simulink model "mainV03_56"  (R2016b)
settings: Solver=FixedStepAuto  StartTime=0.0  StopTime=inf  FixedStep=Ts  MaxStep=0.2  RelTol=1e-2
undefined symbols (not defined in the file): checks, datetime, decyear, delta_e, deltae_degrees, deltafl_degrees, deltafr_degrees, deltar_degrees, deltat_1, deltat_2, deltat_3, deltat_4, deltat_5, Earth, F, ft, groundReaction, initialValues, juliandate, LD, leapyear, Light, m, MIL, Newton, Raphson, s, sigbuilder_block, Ts, WGS84
libraries: simulink x68, aerolibutil x17, aerolibtransform2 x15, simulink_extras x13, aerolibasang x5, aerolib6dofsys x5, aerolib6dof2 x4, aerolibwind2 x3, aerolibbdyn x3, vrlib x3, aerolibconvert2 x3, aerolibactuator x2
(part 7 of 10)

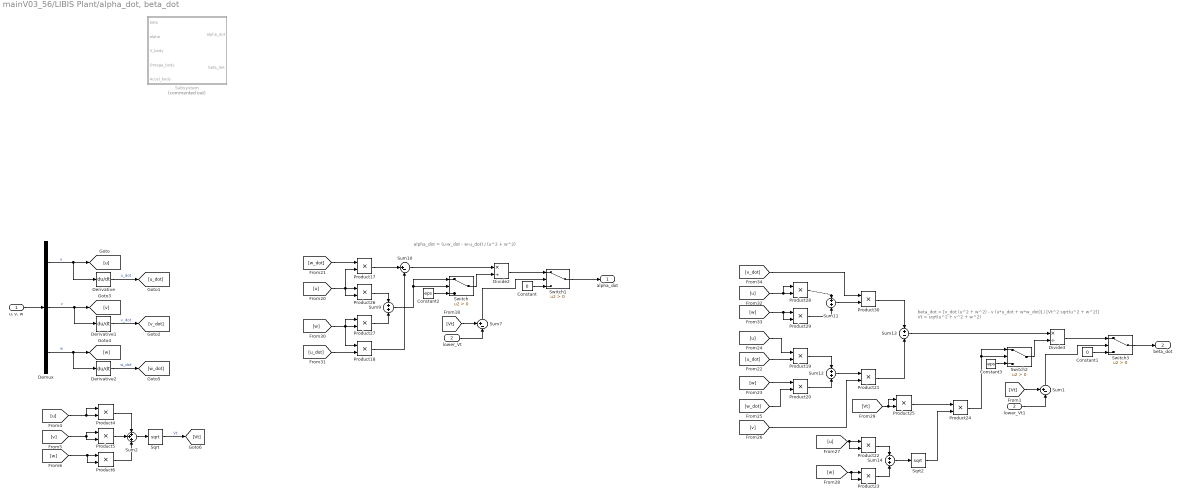
== system mainV03_56/LIBIS Plant/alpha_dot, beta_dot ==
  note: beta_dot = [v_dot (u^2 + w^2) - v (u*u_dot + w*w_dot)] / [Vt^2 sqrt(u^2 + w^2)]
      | Vt = sqrt(u^2 + v^2 + w^2)
  note: alpha_dot = (u·w_dot - w·u_dot) / (u^2 + w^2)
  "u, v, w" : Inport  Unit=meter/s
  lower_Vt : Inport  Port=2
  Constant : Constant  Value=0
  Constant1 : Constant  Value=0
  Constant2 : Constant  Value=eps
  Constant3 : Constant  Value=eps
  Demux : Demux  Outputs=3
  Derivative : Derivative
  Derivative1 : Derivative
  Derivative2 : Derivative
  Divide2 : Product  Inputs=*/
  Divide3 : Product  Inputs=*/
  Product{4..6,17..30} (17 alike) : Product
  Sqrt : Sqrt  SaturateOnIntegerOverflow=on
  Sqrt2 : Sqrt  SaturateOnIntegerOverflow=on
  Subsystem : Subsystem  Commented=on
  Sum1 : Sum  Inputs=+-|
  Sum10 : Sum  Inputs=|+-
  Sum{9,11..12,14} (4 alike) : Sum  Inputs=+|+
  Sum13 : Sum  Inputs=+|-
  Sum2 : Sum  Inputs=+++
  Sum7 : Sum  Inputs=+-|
  Switch{,1..3} (4 alike) : Switch  Criteria=u2 > Threshold
  lower_Vt1 : InportShadow  Port=2
  alpha_dot : Outport  Unit=rad/s
  beta_dot : Outport  Port=2
  wires:
  "u, v, w"/1 -> Demux/1
  Demux/1 -> Derivative/1, [u]  "u"
  Demux/2 -> Derivative1/1, [v]  "v"
  Demux/3 -> Derivative2/1, [w]  "w"
  [u] -> Product4/1, Product4/2
  [w] -> Product6/2, Product6/1
  [v] -> Product5/1, Product5/2
  Product4/1 -> Sum2/1
  Product6/1 -> Sum2/3
  Product5/1 -> Sum2/2
  Sum2/1 -> Sqrt/1
  Sqrt/1 -> [Vt]  "Vt"
  Derivative2/1 -> [w_dot]  "w_dot"
  Derivative/1 -> [u_dot]  "u_dot"
  Derivative1/1 -> [v_dot]  "v_dot"
  Sum7/1 -> Switch1/2
  [Vt] -> Sum7/1
  lower_Vt/1 -> Sum7/2
  [w_dot] -> Product17/1
  [u] -> Product17/2, Product26/2, Product26/1
  [w] -> Product27/1, Product27/2, Product18/1
  [u_dot] -> Product18/2
  Product26/1 -> Sum9/1
  Product27/1 -> Sum9/2
  Product17/1 -> Sum10/1
  Product18/1 -> Sum10/2
  Sum10/1 -> Divide2/1
  [u] -> Product28/1, Product28/2
  [w] -> Product29/2, Product29/1
  Product28/1 -> Sum11/1
  Product29/1 -> Sum11/2
  Sum11/1 -> Product30/2
  [v_dot] -> Product30/1
  [u_dot] -> Product19/2
  [w] -> Product20/1
  Product19/1 -> Sum12/1
  Product20/1 -> Sum12/2
  Sum12/1 -> Product21/1
  [u] -> Product19/1
  [w_dot] -> Product20/2
  [v] -> Product21/2
  Product30/1 -> Sum13/1
  Product21/1 -> Sum13/2
  Sum13/1 -> Divide3/1
  Product22/1 -> Sum14/1
  Product23/1 -> Sum14/2
  [u] -> Product22/2, Product22/1
  [w] -> Product23/2, Product23/1
  [Vt] -> Product25/1, Product25/2
  Product25/1 -> Product24/1
  Sum14/1 -> Sqrt2/1
  Sqrt2/1 -> Product24/2
  Switch/1 -> Divide2/2
  Sum9/1 -> Switch/2, Switch/1
  Constant2/1 -> Switch/3
  Switch2/1 -> Divide3/2
  Product24/1 -> Switch2/2, Switch2/1
  Constant3/1 -> Switch2/3
  Switch3/1 -> beta_dot/1
  Divide2/1 -> Switch1/1
  Switch1/1 -> alpha_dot/1
  Constant/1 -> Switch1/3
  Sum1/1 -> Switch3/2
  Constant1/1 -> Switch3/3
  Divide3/1 -> Switch3/1
  [Vt] -> Sum1/1
  lower_Vt1/1 -> Sum1/2

== system mainV03_56/Pilot Commands/  ==

== system mainV03_56/Pilot Commands/  ==

== system mainV03_56/Pilot Commands/Airspeed Indicator1 ==

== system mainV03_56/Pilot Commands/Altimeter1 ==

== system mainV03_56/Pilot Commands/Artificial Horizon1 ==

== system mainV03_56/Pilot Commands/Buttons to Switches ==
  Buttons : Inport
  Clock : simulink_extras/Flip Flops/Clock  period=2*Ts
  Data Type Conversion : DataTypeConversion  OutDataTypeStr=double
  Data Type Conversion1 : DataTypeConversion  OutDataTypeStr=boolean
  Demux : Demux  Outputs=12
  Hit Crossing : HitCross  HitCrossingOffset=0.5  HitCrossingDirection=rising
  J-K Flip-Flop {1..12} (12 alike) : simulink_extras/Flip Flops/J-K Flip-Flop  initial_condition=0
  Memory : Memory
  Mux : Mux  Inputs=12
  Sum : Sum  Inputs=|++
  Terminator{,1..11} (12 alike) : Terminator
  Switches : Outport
  wires:
  Hit Crossing/1 -> Memory/1, Sum/1
  Buttons/1 -> Data Type Conversion/1
  J-K Flip-Flop 3/2 -> Terminator/1
  Data Type Conversion1/1 -> Demux/1
  Data Type Conversion/1 -> Hit Crossing/1
  Sum/1 -> Data Type Conversion1/1
  Memory/1 -> Sum/2
  J-K Flip-Flop 6/2 -> Terminator1/1
  J-K Flip-Flop 7/2 -> Terminator2/1
  J-K Flip-Flop 10/2 -> Terminator3/1
  J-K Flip-Flop 2/2 -> Terminator4/1
  J-K Flip-Flop 5/2 -> Terminator5/1
  J-K Flip-Flop 8/2 -> Terminator6/1
  J-K Flip-Flop 11/2 -> Terminator7/1
  Clock/1 -> J-K Flip-Flop 9/2, J-K Flip-Flop 12/2, J-K Flip-Flop 4/2, J-K Flip-Flop 1/2, J-K Flip-Flop 2/2, J-K Flip-Flop 5/2, J-K Flip-Flop 11/2, J-K Flip-Flop 8/2, J-K Flip-Flop 3/2, J-K Flip-Flop 10/2, J-K Flip-Flop 7/2, J-K Flip-Flop 6/2
  J-K Flip-Flop 1/2 -> Terminator8/1
  J-K Flip-Flop 4/2 -> Terminator9/1
  J-K Flip-Flop 9/2 -> Terminator10/1
  J-K Flip-Flop 12/2 -> Terminator11/1
  Demux/2 -> J-K Flip-Flop 2/3, J-K Flip-Flop 2/1
  Demux/1 -> J-K Flip-Flop 1/3, J-K Flip-Flop 1/1
  Demux/3 -> J-K Flip-Flop 3/1, J-K Flip-Flop 3/3
  Demux/12 -> J-K Flip-Flop 12/1, J-K Flip-Flop 12/3
  Demux/11 -> J-K Flip-Flop 11/1, J-K Flip-Flop 11/3
  Demux/10 -> J-K Flip-Flop 10/1, J-K Flip-Flop 10/3
  Demux/9 -> J-K Flip-Flop 9/1, J-K Flip-Flop 9/3
  Demux/4 -> J-K Flip-Flop 4/3, J-K Flip-Flop 4/1
  Demux/5 -> J-K Flip-Flop 5/3, J-K Flip-Flop 5/1
  Demux/8 -> J-K Flip-Flop 8/1, J-K Flip-Flop 8/3
  Demux/6 -> J-K Flip-Flop 6/3, J-K Flip-Flop 6/1
  Demux/7 -> J-K Flip-Flop 7/1, J-K Flip-Flop 7/3
  J-K Flip-Flop 1/1 -> Mux/1
  J-K Flip-Flop 12/1 -> Mux/12
  J-K Flip-Flop 11/1 -> Mux/11
  J-K Flip-Flop 10/1 -> Mux/10
  J-K Flip-Flop 9/1 -> Mux/9
  J-K Flip-Flop 8/1 -> Mux/8
  J-K Flip-Flop 7/1 -> Mux/7
  J-K Flip-Flop 4/1 -> Mux/4
  J-K Flip-Flop 5/1 -> Mux/5
  J-K Flip-Flop 6/1 -> Mux/6
  J-K Flip-Flop 2/1 -> Mux/2
  J-K Flip-Flop 3/1 -> Mux/3
  Mux/1 -> Switches/1

== system mainV03_56/Pilot Commands/Climb Rate Indicator1 ==

== system mainV03_56/Pilot Commands/Heading Indicator1 ==

== system mainV03_56/Pilot Commands/If Action Subsystem ==
  Action Port : ActionPort  ActionType=then
  Joystick Input : vrlib/Joystick Input  joyid=1  adjustports=on  forcefeed=off
  Axes : Outport
  Buttons : Outport  Port=2
  wires:
  Joystick Input/1 -> Axes/1
  Joystick Input/2 -> Buttons/1

== system mainV03_56/Pilot Commands/Remaining Capacity Indicator1 ==

== system mainV03_56/Pilot Commands/Signal Builder ==
  Demux : Demux  Tag=STV Demux  Outputs=6
  FromWs : FromWorkspace  Tag=STV FromWs  VariableName=tuvar  SampleTime=0
      SigBuilderData=|
      | common.afterFinalStr = 'Extrapolate'
      | common.sampleTime = 0
      | dataSet.timeRange = [0 500]
      | dataSet.name = 'Group 1'
      | sbobj.Groups.Name = 'Group 1'
      | sbobj.Groups.Signals(1).Name = 'Roll'
      | sbobj.Groups.Signals(1).XData = [0 500]
      | sbobj.Groups.Signals(1).YData = [0 0]
      | sbobj.Groups.Signals(2).Name = 'Pitch'
      | sbobj.Groups.Signals(2).XData = [0 500]
      | sbobj.Groups.Signals(2).YData = [0 0]
      | sbobj.Groups.Signals(3).Name = 'Yaw'
      | sbobj.Groups.Signals(3).XData = [0 500]
      | sbobj.Groups.Signals(3).YData = [0 0]
      | sbobj.Groups.Signals(4).Name = 'Altitude'
      | sbobj.Groups.Signals(4).XData = [0 500]
      | sbobj.Groups.Signals(4).YData = [0 0]
      | sbobj.Groups.Signals(5).Name = 'Throttle1'
      | sbobj.Groups.Signals(5).XData = [0 500]
      | sbobj.Groups.Signals(5).YData = [0 0]
      | sbobj.Groups.Signals(6).Name = 'flightCondition'
      | sbobj.Groups.Signals(6).XData = [0 500]
      | sbobj.Groups.Signals(6).YData = [0 0]
      | sbobj.Groups.TimeRange = [0 500]
  Roll : Outport  Tag=STV Outport
  Pitch : Outport  Tag=STV Outport  Port=2
  Yaw : Outport  Tag=STV Outport  Port=3
  Altitude : Outport  Tag=STV Outport  Port=4
  Throttle1 : Outport  Tag=STV Outport  Port=5
  flightCondition : Outport  Tag=STV Outport  Port=6
  wires:
  FromWs/1 -> Demux/1
  Demux/1 -> Roll/1
  Demux/2 -> Pitch/1
  Demux/3 -> Yaw/1
  Demux/4 -> Altitude/1
  Demux/5 -> Throttle1/1
  Demux/6 -> flightCondition/1

== system mainV03_56/Sensors/Feedthrough Sensors ==
  States : Inport  OutDataTypeStr=Bus: plantDataBus
  Environment : Inport  Port=2  OutDataTypeStr=Bus: envDataBus
  Bus Creator2 : BusCreator  Inputs='LLAMeas','X_nedMeas','VearthMeas','AccelMeas_body','OmegaMeas_body','DCMMeas_body_earth','EulerMeas','VaeroMeas_body','alphaMeas','betaMeas','CGMeas','remainingCapacityMeas'  OutDataTypeStr=Bus: SensorsBus  NonVirtualBus=on
  CPU : Subsystem
  Environment_1 : InportShadow  Port=2  OutDataTypeStr=Bus: envDataBus
  GPS : Subsystem
  IMU : Subsystem
  Pitot : Subsystem
  Veleta : Subsystem
  Sensors : Outport  OutDataTypeStr=Bus: SensorsBus
  wires:
  Environment/1 -> IMU/2(Environment)
  IMU/4(EulerMeas) -> Bus Creator2/7  "EulerMeas"
  Bus Creator2/1 -> Sensors/1  "Sensors"
  CPU/1(CGMeas) -> Bus Creator2/11  "CGMeas"
  GPS/2(X_nedMeas) -> Bus Creator2/2  "X_nedMeas"
  States/1 -> IMU/1(States), GPS/1(States), Pitot/1(States), CPU/1(States), Veleta/1(States)
  IMU/2(OmegaMeas_body) -> Bus Creator2/5  "OmegaMeas_body"
  IMU/1(AccelMeas_body) -> Bus Creator2/4  "AccelMeas_body"
  GPS/1(LLAMeas) -> Bus Creator2/1  "LLAMeas"
  Veleta/1(alphaMeas) -> Bus Creator2/9  "alphaMeas"
  Environment_1/1 -> Pitot/2(Environment)
  Veleta/2(betaMeas) -> Bus Creator2/10  "betaMeas"
  Pitot/1(VaeroMeas_body) -> Bus Creator2/8  "VaeroMeas_body"
  CPU/2(remainingCapacityMeas) -> Bus Creator2/12  "remainingCapacityMeas"
  GPS/3(VearthMeas) -> Bus Creator2/3  "VearthMeas"
  IMU/3(DCMMeas_body_earth) -> Bus Creator2/6  "DCMMeas_body_earth"

== system mainV03_56/Sensors/Noisy Sensors ==
  States : Inport  OutDataTypeStr=Bus: plantDataBus
  Environment : Inport  Port=2  OutDataTypeStr=Bus: envDataBus
  Bus Creator2 : BusCreator  Inputs='LLAMeas','X_nedMeas','VearthMeas','AccelMeas_body','OmegaMeas_body','DCMMeas_body_earth','EulerMeas','VaeroMeas_body','alphaMeas','betaMeas','CGMeas','remainingCapacityMeas'  OutDataTypeStr=Bus: SensorsBus  NonVirtualBus=on
  CPU (Feedthough) : Subsystem
  Environment_1 : InportShadow  Port=2  OutDataTypeStr=Bus: envDataBus
  GPS (Feedthough) : Subsystem
  IMU : Subsystem
  Pitot (Feedthough) : Subsystem
  Veleta (Feedthough) : Subsystem
  Sensors : Outport  OutDataTypeStr=Bus: SensorsBus
  wires:
  Environment/1 -> IMU/2(Environment)
  IMU/4(EulerMeas) -> Bus Creator2/7  "EulerMeas"
  Bus Creator2/1 -> Sensors/1  "Sensors"
  CPU (Feedthough)/1(CGMeas) -> Bus Creator2/11  "CGMeas"
  GPS (Feedthough)/2(X_nedMeas) -> Bus Creator2/2  "X_nedMeas"
  States/1 -> GPS (Feedthough)/1(States), IMU/1(States), Pitot (Feedthough)/1(States), CPU (Feedthough)/1(States), Veleta (Feedthough)/1(States)
  IMU/2(OmegaMeas_body) -> Bus Creator2/5  "OmegaMeas_body"
  IMU/1(AccelMeas_body) -> Bus Creator2/4  "AccelMeas_body"
  GPS (Feedthough)/1(LLAMeas) -> Bus Creator2/1  "LLAMeas"
  Veleta (Feedthough)/1(alphaMeas) -> Bus Creator2/9  "alphaMeas"
  Environment_1/1 -> Pitot (Feedthough)/2(Environment)
  Veleta (Feedthough)/2(betaMeas) -> Bus Creator2/10  "betaMeas"
  Pitot (Feedthough)/1(VaeroMeas_body) -> Bus Creator2/8  "VaeroMeas_body"
  CPU (Feedthough)/2(remainingCapacityMeas) -> Bus Creator2/12  "remainingCapacityMeas"
  GPS (Feedthough)/3(VearthMeas) -> Bus Creator2/3  "VearthMeas"
  IMU/3(DCMMeas_body_earth) -> Bus Creator2/6  "DCMMeas_body_earth"

== system mainV03_56/Visualization/Airspeed Indicator ==

== system mainV03_56/Visualization/Altimeter ==

== system mainV03_56/Visualization/Artificial Horizon ==

== system mainV03_56/Visualization/Axes to VR Axes ==
  Xe : Inport
  Concatenate : Concatenate  NumInputs=3
  Constant : Constant  Value=1.01
  Demux : Demux  Outputs=3
  Sum : Sum  Inputs=|++
  rad-->deg : Gain  Gain=-1  SaturateOnIntegerOverflow=on  OutDataTypeStr=Inherit: Same as input  ParamDataTypeStr=Inherit: Same as input
  rad-->deg1 : Gain  Gain=-1  SaturateOnIntegerOverflow=on  OutDataTypeStr=Inherit: Same as input  ParamDataTypeStr=Inherit: Same as input
  Xe VR : Outport
  wires:
  Xe/1 -> Demux/1
  Concatenate/1 -> Xe VR/1
  rad-->deg1/1 -> Concatenate/2
  rad-->deg/1 -> Concatenate/1
  Demux/1 -> Concatenate/3
  Demux/2 -> rad-->deg/1
  Constant/1 -> Sum/2
  Demux/3 -> Sum/1
  Sum/1 -> rad-->deg1/1

== system mainV03_56/Visualization/Climb Rate Indicator ==

== system mainV03_56/Visualization/Heading Indicator ==

== system mainV03_56/Visualization/Remaining Capacity Indicator ==

== system mainV03_56/Visualization/Subsystem ==
  "X_ned " : Inport
  Euler_angles : Inport  Port=2
  V_body : Inport  Port=3
  V_ned : Inport  Port=4
  Angle Conversion : aerolibconvert2/Angle Conversion  IU=rad  OU=deg
  Angle Conversion1 : aerolibconvert2/Angle Conversion  IU=rad  OU=deg
  Climbrate : Selector  IndexMode=Zero-based  InputPortWidth=3  IndexOptions=Index vector (dialog)  Indices=2  OutputSizes=1
  Concatenate : Concatenate
  Dot Product : DotProduct  SaturateOnIntegerOverflow=on  OutDataTypeStr=Inherit: Inherit via internal rule
  Flightpath Angle : Subsystem
  Heading : Selector  IndexMode=Zero-based  InputPortWidth=3  IndexOptions=Index vector (dialog)  Indices=2  OutputSizes=1
  Height : Selector  IndexMode=Zero-based  InputPortWidth=3  IndexOptions=Index vector (dialog)  Indices=2  OutputSizes=1
  Length Conversion : aerolibconvert2/Length Conversion  IU=m  OU=ft
  Roll Angle : Selector  IndexMode=Zero-based  InputPortWidth=3  IndexOptions=Index vector (dialog)  Indices=0  OutputSizes=1
  Velocity Conversion : aerolibconvert/Velocity Conversion  IU=m/s  OU=kts
  Velocity Conversion1 : aerolibconvert/Velocity Conversion  IU=m/s  OU=ft/s
  rad-->deg1 : Gain  Gain=-1  SaturateOnIntegerOverflow=on  OutDataTypeStr=Inherit: Same as input  ParamDataTypeStr=Inherit: Same as input
  rad-->deg2 : Gain  Gain=-1  SaturateOnIntegerOverflow=on  OutDataTypeStr=Inherit: Same as input  ParamDataTypeStr=Inherit: Same as input
  rad-->deg3 : Gain  Gain=60  SaturateOnIntegerOverflow=on  OutDataTypeStr=Inherit: Same as input  ParamDataTypeStr=Inherit: Same as input
  vt : Sqrt  SaturateOnIntegerOverflow=on
  Airspeed (kts) : Outport
  Height (ft) : Outport  Port=2
  Roll Flightpath (deg) : Outport  Port=3
  Climb Rate (ft/min) : Outport  Port=4
  Heading (deg) : Outport  Port=5
  wires:
  Velocity Conversion1/1 -> rad-->deg3/1
  rad-->deg3/1 -> Climb Rate (ft/min)/1
  V_ned/1 -> Flightpath Angle/1(Ve), Climbrate/1
  Flightpath Angle/1(gamma) -> Concatenate/2
  rad-->deg2/1 -> Velocity Conversion1/1
  Length Conversion/1 -> Height (ft)/1
  Angle Conversion1/1 -> Roll Flightpath (deg)/1
  Height/1 -> rad-->deg1/1
  Angle Conversion/1 -> Heading (deg)/1  "Heading"
  Heading/1 -> Angle Conversion/1
  Velocity Conversion/1 -> Airspeed (kts)/1
  Dot Product/1 -> vt/1
  Roll Angle/1 -> Concatenate/1
  V_body/1 -> Dot Product/2, Dot Product/1
  Concatenate/1 -> Angle Conversion1/1
  vt/1 -> Velocity Conversion/1
  Climbrate/1 -> rad-->deg2/1
  rad-->deg1/1 -> Length Conversion/1
  Euler_angles/1 -> Roll Angle/1, Heading/1
  "X_ned "/1 -> Height/1

== system mainV03_56/Environment/Terrain/Reaction ==
  X : Inport
  V : Inport  Port=2
  -D1 : Gain  Gain=-groundReaction.D
  -K2 : Gain  Gain=-groundReaction.K
  Constant3 : Constant  Value=0
  Constant4 : Constant  Value=0
  Constant5 : Constant  Value=0
  Mux1 : Mux  Inputs=3
  Product1 : Product
  Sel5 : Selector  InputPortWidth=3  IndexOptions=Index vector (dialog)  Indices=3  OutputSizes=1
  Sel6 : Selector  InputPortWidth=3  IndexOptions=Index vector (dialog)  Indices=3  OutputSizes=1
  Sqrt1 : Sqrt  SaturateOnIntegerOverflow=on
  Sum4 : Sum  Inputs=|++
  Sum5 : Sum  Inputs=-+
  Switch3 : Switch  Criteria=u2 > Threshold
  Ze2height1 : UnaryMinus
  Ze_dot2height_dot3 : UnaryMinus
  height2d2 : UnaryMinus
  height2d3 : UnaryMinus
  hground_value1 : Constant  Value=initialValues.href  OutDataTypeStr=double
  hground1 : Outport  Unit=m
  F_earth : Outport  Port=2
  wires:
  Ze2height1/1 -> Sum5/2  "alt"
  X/1 -> Sel6/1
  Sel6/1 -> Ze2height1/1
  Sel5/1 -> Ze_dot2height_dot3/1
  hground_value1/1 -> Sum5/1
  Constant3/1 -> Switch3/1
  Switch3/1 -> height2d2/1
  height2d2/1 -> Sqrt1/1  "d"
  -K2/1 -> Sum4/1
  Product1/1 -> height2d3/1
  height2d3/1 -> Mux1/3
  Sum5/1 -> hground1/1, -K2/1, Switch3/3, Switch3/2  "z"
  Sqrt1/1 -> Product1/1
  Ze_dot2height_dot3/1 -> -D1/1  "z_dot"
  -D1/1 -> Sum4/2
  Sum4/1 -> Product1/2
  V/1 -> Sel5/1
  Mux1/1 -> F_earth/1  "F_earth"
  Constant5/1 -> Mux1/2
  Constant4/1 -> Mux1/1

== system mainV03_56/Environment/Terrain/Reaction1 ==
  X : Inport
  V : Inport  Port=2
  -D1 : Gain  Gain=-groundReaction.D
  -K2 : Gain  Gain=-groundReaction.K
  Constant3 : Constant  Value=0
  Constant4 : Constant  Value=0
  Constant5 : Constant  Value=0
  Mux1 : Mux  Inputs=3
  Product1 : Product
  Sel5 : Selector  InputPortWidth=3  IndexOptions=Index vector (dialog)  Indices=3  OutputSizes=1
  Sel6 : Selector  InputPortWidth=3  IndexOptions=Index vector (dialog)  Indices=3  OutputSizes=1
  Sqrt1 : Sqrt  SaturateOnIntegerOverflow=on
  Sum4 : Sum  Inputs=|++
  Sum5 : Sum  Inputs=-+
  Switch3 : Switch  Criteria=u2 > Threshold
  Ze2height1 : UnaryMinus
  Ze_dot2height_dot3 : UnaryMinus
  height2d2 : UnaryMinus
  height2d3 : UnaryMinus
  hground_value1 : Constant  Value=initialValues.href  OutDataTypeStr=double
  hground1 : Outport  Unit=m
  F_earth : Outport  Port=2
  wires:
  Ze2height1/1 -> Sum5/2  "alt"
  X/1 -> Sel6/1
  Sel6/1 -> Ze2height1/1
  Sel5/1 -> Ze_dot2height_dot3/1
  hground_value1/1 -> Sum5/1
  Constant3/1 -> Switch3/1
  Switch3/1 -> height2d2/1
  height2d2/1 -> Sqrt1/1  "d"
  -K2/1 -> Sum4/1
  Product1/1 -> height2d3/1
  height2d3/1 -> Mux1/3
  Sum5/1 -> hground1/1, -K2/1, Switch3/3, Switch3/2  "z"
  Sqrt1/1 -> Product1/1
  Ze_dot2height_dot3/1 -> -D1/1  "z_dot"
  -D1/1 -> Sum4/2
  Sum4/1 -> Product1/2
  V/1 -> Sel5/1
  Mux1/1 -> F_earth/1  "F_earth"
  Constant5/1 -> Mux1/2
  Constant4/1 -> Mux1/1

== system mainV03_56/Environment/Terrain/Reaction2 ==
  X : Inport
  V : Inport  Port=2
  -D1 : Gain  Gain=-groundReaction.D
  -K2 : Gain  Gain=-groundReaction.K
  Constant3 : Constant  Value=0
  Constant4 : Constant  Value=0
  Constant5 : Constant  Value=0
  Mux1 : Mux  Inputs=3
  Product1 : Product
  Sel5 : Selector  InputPortWidth=3  IndexOptions=Index vector (dialog)  Indices=3  OutputSizes=1
  Sel6 : Selector  InputPortWidth=3  IndexOptions=Index vector (dialog)  Indices=3  OutputSizes=1
  Sqrt1 : Sqrt  SaturateOnIntegerOverflow=on
  Sum4 : Sum  Inputs=|++
  Sum5 : Sum  Inputs=-+
  Switch3 : Switch  Criteria=u2 > Threshold
  Ze2height1 : UnaryMinus
  Ze_dot2height_dot3 : UnaryMinus
  height2d2 : UnaryMinus
  height2d3 : UnaryMinus
  hground_value1 : Constant  Value=initialValues.href  OutDataTypeStr=double
  hground1 : Outport  Unit=m
  F_earth : Outport  Port=2
  wires:
  Ze2height1/1 -> Sum5/2  "alt"
  X/1 -> Sel6/1
  Sel6/1 -> Ze2height1/1
  Sel5/1 -> Ze_dot2height_dot3/1
  hground_value1/1 -> Sum5/1
  Constant3/1 -> Switch3/1
  Switch3/1 -> height2d2/1
  height2d2/1 -> Sqrt1/1  "d"
  -K2/1 -> Sum4/1
  Product1/1 -> height2d3/1
  height2d3/1 -> Mux1/3
  Sum5/1 -> hground1/1, -K2/1, Switch3/3, Switch3/2  "z"
  Sqrt1/1 -> Product1/1
  Ze_dot2height_dot3/1 -> -D1/1  "z_dot"
  -D1/1 -> Sum4/2
  Sum4/1 -> Product1/2
  V/1 -> Sel5/1
  Mux1/1 -> F_earth/1  "F_earth"
  Constant5/1 -> Mux1/2
  Constant4/1 -> Mux1/1

== system mainV03_56/FCS/Fixed-Wing - Cruise/Slider ==

== system mainV03_56/FCS/Fixed-Wing - Cruise/Slider10 ==

== system mainV03_56/FCS/Fixed-Wing - Cruise/Slider11 ==

== system mainV03_56/FCS/Fixed-Wing - Cruise/Slider12 ==

== system mainV03_56/FCS/Fixed-Wing - Cruise/Slider13 ==

== system mainV03_56/FCS/Fixed-Wing - Cruise/Slider6 ==

== system mainV03_56/FCS/Fixed-Wing - Cruise/Slider7 ==

== system mainV03_56/FCS/Fixed-Wing - Cruise/Slider8 ==

== system mainV03_56/FCS/Fixed-Wing - Cruise/Slider9 ==

== system mainV03_56/FCS/Fixed-Wing Climb/Slider ==

== system mainV03_56/FCS/Fixed-Wing Climb/Slider10 ==

== system mainV03_56/FCS/Fixed-Wing Climb/Slider11 ==

== system mainV03_56/FCS/Fixed-Wing Climb/Slider12 ==

== system mainV03_56/FCS/Fixed-Wing Climb/Slider13 ==

== system mainV03_56/FCS/Fixed-Wing Climb/Slider6 ==

== system mainV03_56/FCS/Fixed-Wing Climb/Slider7 ==

== system mainV03_56/FCS/Fixed-Wing Climb/Slider8 ==

== system mainV03_56/FCS/Fixed-Wing Climb/Slider9 ==

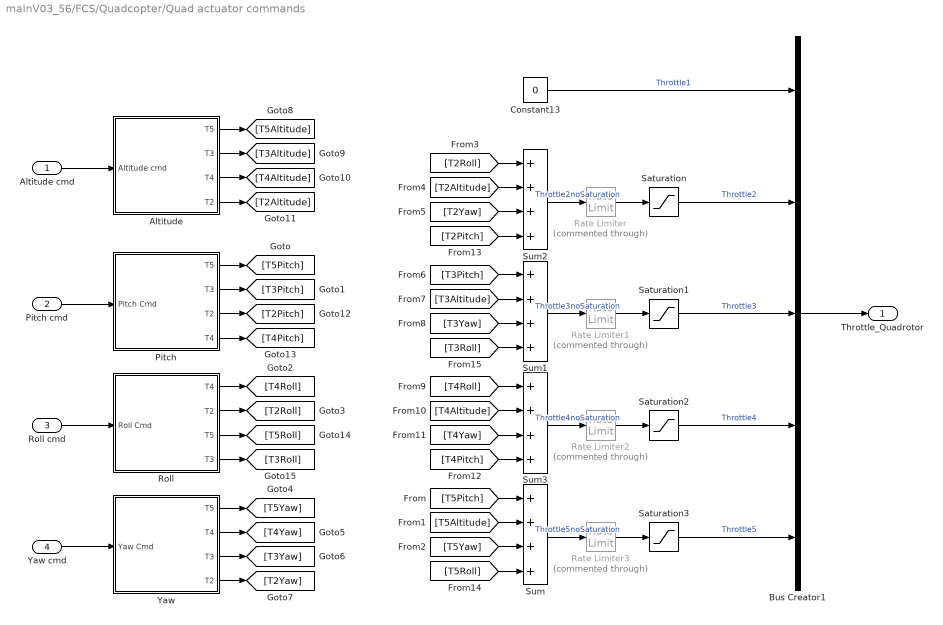
== system mainV03_56/FCS/Quadcopter/Quad actuator commands ==
  Altitude cmd : Inport
  Pitch cmd : Inport  Port=2
  Roll cmd : Inport  Port=3
  Yaw cmd : Inport  Port=4
  Altitude : Subsystem
  Bus Creator1 : BusCreator  Inputs='Throttle1','Throttle2','Throttle3','Throttle4','Throttle5'  OutDataTypeStr=Bus: ThrottleBus  NonVirtualBus=on
  Constant13 : Constant  Value=0
  Pitch : Subsystem
  Rate Limiter{,1..3} (4 alike) : RateLimiter  Commented=through  RisingSlewLimit=0.5  FallingSlewLimit=-0.5  SampleTimeMode=inherited
  Roll : Subsystem
  Saturation{,1..3} (4 alike) : Saturate  UpperLimit=1  LowerLimit=0
  Sum{,1..3} (4 alike) : Sum  Inputs=++++
  Yaw : Subsystem
  Throttle_Quadrotor : Outport  OutDataTypeStr=Bus: ThrottleBus
  wires:
  [T4Yaw] -> Sum3/3
  [T4Altitude] -> Sum3/2
  [T4Roll] -> Sum3/1
  [T3Yaw] -> Sum1/3
  [T3Altitude] -> Sum1/2
  [T3Pitch] -> Sum1/1
  [T2Yaw] -> Sum2/3
  [T2Altitude] -> Sum2/2
  [T2Roll] -> Sum2/1
  [T5Yaw] -> Sum/3
  [T5Altitude] -> Sum/2
  [T5Pitch] -> Sum/1
  Altitude/4(T2) -> [T2Altitude]
  Altitude/3(T4) -> [T4Altitude]
  Altitude/2(T3) -> [T3Altitude]
  Altitude/1(T5) -> [T5Altitude]
  Yaw/4(T2) -> [T2Yaw]
  Yaw/1(T5) -> [T5Yaw]
  Roll/2(T2) -> [T2Roll]
  Roll/1(T4) -> [T4Roll]
  Pitch/2(T3) -> [T3Pitch]
  Pitch/1(T5) -> [T5Pitch]
  Bus Creator1/1 -> Throttle_Quadrotor/1
  Pitch cmd/1 -> Pitch/1(Pitch Cmd)
  Roll cmd/1 -> Roll/1(Roll Cmd)
  Altitude cmd/1 -> Altitude/1(Altitude cmd)
  Yaw/2(T4) -> [T4Yaw]
  Yaw/3(T3) -> [T3Yaw]
  Yaw cmd/1 -> Yaw/1(Yaw Cmd)
  Pitch/3(T2) -> [T2Pitch]
  Pitch/4(T4) -> [T4Pitch]
  [T4Pitch] -> Sum3/4
  [T2Pitch] -> Sum2/4
  Roll/3(T5) -> [T5Roll]
  Roll/4(T3) -> [T3Roll]
  [T5Roll] -> Sum/4
  [T3Roll] -> Sum1/4
  Sum2/1 -> Rate Limiter/1  "Throttle2noSaturation"
  Sum/1 -> Rate Limiter3/1  "Throttle5noSaturation"
  Sum3/1 -> Rate Limiter2/1  "Throttle4noSaturation"
  Sum1/1 -> Rate Limiter1/1  "Throttle3noSaturation"
  Constant13/1 -> Bus Creator1/1  "Throttle1"
  Saturation/1 -> Bus Creator1/2  "Throttle2"
  Saturation1/1 -> Bus Creator1/3  "Throttle3"
  Saturation2/1 -> Bus Creator1/4  "Throttle4"
  Saturation3/1 -> Bus Creator1/5  "Throttle5"
  Rate Limiter/1 -> Saturation/1
  Rate Limiter1/1 -> Saturation1/1
  Rate Limiter2/1 -> Saturation2/1
  Rate Limiter3/1 -> Saturation3/1

== system mainV03_56/FCS/Quadcopter/Slider ==

== system mainV03_56/FCS/Quadcopter/Slider10 ==

== system mainV03_56/FCS/Quadcopter/Slider11 ==

== system mainV03_56/FCS/Quadcopter/Slider12 ==

== system mainV03_56/FCS/Quadcopter/Slider13 ==

== system mainV03_56/FCS/Quadcopter/Slider6 ==

== system mainV03_56/FCS/Quadcopter/Slider7 ==

== system mainV03_56/FCS/Quadcopter/Slider8 ==

== system mainV03_56/FCS/Quadcopter/Slider9 ==

== system mainV03_56/FCS/Quadcopter --> Fixed-Wing/Quad actuator commands ==
  Altitude cmd : Inport
  Pitch cmd : Inport  Port=2
  Roll cmd : Inport  Port=3
  Yaw cmd : Inport  Port=4
  Throttle1 : Inport  Port=5
  Altitude : Subsystem
  Bus Creator1 : BusCreator  Inputs='Throttle1','Throttle2','Throttle3','Throttle4','Throttle5'  OutDataTypeStr=Bus: ThrottleBus  NonVirtualBus=on
  Pitch : Subsystem
  Rate Limiter{,1..3} (4 alike) : RateLimiter  Commented=through  RisingSlewLimit=0.5  FallingSlewLimit=-0.5  SampleTimeMode=inherited
  Roll : Subsystem
  Saturation{,1..3} (4 alike) : Saturate  UpperLimit=1  LowerLimit=0
  Sum{,1..3} (4 alike) : Sum  Inputs=++++
  Yaw : Subsystem
  Throttle_Quadrotor : Outport  OutDataTypeStr=Bus: ThrottleBus
  wires:
  [T4Yaw] -> Sum3/3
  [T4Altitude] -> Sum3/2
  [T4Roll] -> Sum3/1
  [T3Yaw] -> Sum1/3
  [T3Altitude] -> Sum1/2
  [T3Pitch] -> Sum1/1
  [T2Yaw] -> Sum2/3
  [T2Altitude] -> Sum2/2
  [T2Roll] -> Sum2/1
  [T5Yaw] -> Sum/3
  [T5Altitude] -> Sum/2
  [T5Pitch] -> Sum/1
  Altitude/4(T2) -> [T2Altitude]
  Altitude/3(T4) -> [T4Altitude]
  Altitude/2(T3) -> [T3Altitude]
  Altitude/1(T5) -> [T5Altitude]
  Yaw/4(T2) -> [T2Yaw]
  Yaw/1(T5) -> [T5Yaw]
  Roll/2(T2) -> [T2Roll]
  Roll/1(T4) -> [T4Roll]
  Pitch/2(T3) -> [T3Pitch]
  Pitch/1(T5) -> [T5Pitch]
  Bus Creator1/1 -> Throttle_Quadrotor/1
  Pitch cmd/1 -> Pitch/1(Pitch Cmd)
  Roll cmd/1 -> Roll/1(Roll Cmd)
  Altitude cmd/1 -> Altitude/1(Altitude cmd)
  Yaw/2(T4) -> [T4Yaw]
  Yaw/3(T3) -> [T3Yaw]
  Yaw cmd/1 -> Yaw/1(Yaw Cmd)
  Pitch/3(T2) -> [T2Pitch]
  Pitch/4(T4) -> [T4Pitch]
  [T4Pitch] -> Sum3/4
  [T2Pitch] -> Sum2/4
  Roll/3(T5) -> [T5Roll]
  Roll/4(T3) -> [T3Roll]
  [T5Roll] -> Sum/4
  [T3Roll] -> Sum1/4
  Sum2/1 -> Rate Limiter/1  "Throttle2noSaturation"
  Sum/1 -> Rate Limiter3/1  "Throttle5noSaturation"
  Sum3/1 -> Rate Limiter2/1  "Throttle4noSaturation"
  Sum1/1 -> Rate Limiter1/1  "Throttle3noSaturation"
  Throttle1/1 -> Bus Creator1/1  "Throttle1"
  Saturation/1 -> Bus Creator1/2  "Throttle2"
  Saturation1/1 -> Bus Creator1/3  "Throttle3"
  Saturation2/1 -> Bus Creator1/4  "Throttle4"
  Saturation3/1 -> Bus Creator1/5  "Throttle5"
  Rate Limiter/1 -> Saturation/1
  Rate Limiter1/1 -> Saturation1/1
  Rate Limiter2/1 -> Saturation2/1
  Rate Limiter3/1 -> Saturation3/1

== system mainV03_56/FCS/Quadcopter --> Fixed-Wing/Slider10 ==

== system mainV03_56/FCS/Quadcopter --> Fixed-Wing/Slider11 ==

== system mainV03_56/FCS/Quadcopter --> Fixed-Wing/Slider12 ==

== system mainV03_56/FCS/Quadcopter --> Fixed-Wing/Slider13 ==

== system mainV03_56/FCS/Quadcopter --> Fixed-Wing/Slider9 ==

== system mainV03_56/FCS/TakeOff/Slider ==

== system mainV03_56/FCS/TakeOff/Slider10 ==

== system mainV03_56/FCS/TakeOff/Slider11 ==

== system mainV03_56/FCS/TakeOff/Slider12 ==

== system mainV03_56/FCS/TakeOff/Slider13 ==

== system mainV03_56/FCS/TakeOff/Slider6 ==

== system mainV03_56/FCS/TakeOff/Slider7 ==

== system mainV03_56/FCS/TakeOff/Slider8 ==

== system mainV03_56/FCS/TakeOff/Slider9 ==

== system mainV03_56/LIBIS Plant/Aerodynamics/CD ==
  prelook-ups : Inport
  plantData : Inport  Port=2
  actuators : Inport  Port=3
  Add : Sum  Inputs=+++++++
  Bus Selector : BusSelector  OutputSignals=alpha,alpha_dot,Omega_body.q
  Bus Selector1 : BusSelector  OutputSignals=alpha,beta,alt,xcg,deltae,deltar,deltafr,deltafl
  Bus Selector2 : BusSelector  OutputSignals=deltae,deltafr,deltafl
  CD0 : Interpolation_n-D  NumberOfTableDimensions=8  Table=LD.Stability.CD0  ExtrapMethod=Clip  DiagnosticForOutOfRangeInput=Warning  RequireIndexFractionAsBus=on  ValidIndexMayReachLast=on  InternalRulePriority=Speed
      settings: InputPortMap=u0,u1,u2,u3,u4,u5,u6,u7
  CDalpha : Interpolation_n-D  NumberOfTableDimensions=8  Table=LD.Stability.CDalpha  ExtrapMethod=Clip  DiagnosticForOutOfRangeInput=Warning  RequireIndexFractionAsBus=on  ValidIndexMayReachLast=on  InternalRulePriority=Speed
      settings: InputPortMap=u0,u1,u2,u3,u4,u5,u6,u7
  CDalpha_dot : Interpolation_n-D  NumberOfTableDimensions=8  Table=LD.Stability.CDalpha_dot  ExtrapMethod=Clip  RequireIndexFractionAsBus=on  ValidIndexMayReachLast=on  InternalRulePriority=Speed
      settings: InputPortMap=u0,u1,u2,u3,u4,u5,u6,u7
  CDdeltae : Interpolation_n-D  NumberOfTableDimensions=8  Table=LD.Stability.CDdeltae  ExtrapMethod=Clip  RequireIndexFractionAsBus=on  ValidIndexMayReachLast=on  InternalRulePriority=Speed
      settings: InputPortMap=u0,u1,u2,u3,u4,u5,u6,u7
  CDdeltafr : Interpolation_n-D  NumberOfTableDimensions=8  Table=LD.Stability.CDdeltafr  ExtrapMethod=Clip  RequireIndexFractionAsBus=on  ValidIndexMayReachLast=on  InternalRulePriority=Speed
      settings: InputPortMap=u0,u1,u2,u3,u4,u5,u6,u7
  CDdeltafrl : Interpolation_n-D  NumberOfTableDimensions=8  Table=LD.Stability.CDdeltafl  ExtrapMethod=Clip  RequireIndexFractionAsBus=on  ValidIndexMayReachLast=on  InternalRulePriority=Speed
      settings: InputPortMap=u0,u1,u2,u3,u4,u5,u6,u7
  CDq : Interpolation_n-D  NumberOfTableDimensions=8  Table=LD.Stability.CDq  ExtrapMethod=Clip  RequireIndexFractionAsBus=on  ValidIndexMayReachLast=on  InternalRulePriority=Speed
      settings: InputPortMap=u0,u1,u2,u3,u4,u5,u6,u7
  Product{,1..5} (6 alike) : Product
  CD : Outport
  wires:
  prelook-ups/1 -> Bus Selector1/1
  CD0/1 -> Add/1
  Add/1 -> CD/1
  plantData/1 -> Bus Selector/1
  actuators/1 -> Bus Selector2/1
  Product/1 -> Add/2
  Bus Selector/1 -> Product/2  "<alpha>"
  Bus Selector2/1 -> Product3/2  "<deltae>"
  CDdeltae/1 -> Product3/1
  Product3/1 -> Add/5
  Product2/1 -> Add/4
  Product1/1 -> Add/3
  CDalpha_dot/1 -> Product1/1
  CDq/1 -> Product2/1
  Bus Selector/3 -> Product2/2  "<q>"
  Bus Selector/2 -> Product1/2  "<alpha_dot>"
  Bus Selector1/8 -> CD0/8, CDalpha/8, CDq/8, CDdeltafrl/8, CDdeltafr/8, CDdeltae/8, CDalpha_dot/8  "<deltafl>"
  Bus Selector1/7 -> CD0/7, CDalpha/7, CDq/7, CDdeltafrl/7, CDdeltafr/7, CDdeltae/7, CDalpha_dot/7  "<deltafr>"
  Bus Selector1/6 -> CD0/6, CDalpha/6, CDq/6, CDdeltafrl/6, CDdeltafr/6, CDdeltae/6, CDalpha_dot/6  "<deltar>"
  Bus Selector1/5 -> CD0/5, CDalpha/5, CDq/5, CDdeltafrl/5, CDdeltafr/5, CDdeltae/5, CDalpha_dot/5  "<deltae>"
  Bus Selector1/3 -> CD0/3, CDalpha/3, CDq/3, CDdeltafrl/3, CDdeltafr/3, CDdeltae/3, CDalpha_dot/3  "<alt>"
  Bus Selector1/4 -> CD0/4, CDalpha/4, CDq/4, CDdeltafrl/4, CDdeltafr/4, CDdeltae/4, CDalpha_dot/4  "<xcg>"
  Bus Selector1/1 -> CD0/1, CDalpha/1, CDdeltafrl/1, CDdeltafr/1, CDdeltae/1, CDq/1, CDalpha_dot/1  "<alpha>"
  Bus Selector2/3 -> Product5/2  "<deltafl>"
  CDdeltafrl/1 -> Product5/1
  Product5/1 -> Add/7
  Product4/1 -> Add/6
  CDdeltafr/1 -> Product4/1
  Bus Selector2/2 -> Product4/2  "<deltafr>"
  Bus Selector1/2 -> CD0/2, CDdeltafrl/2, CDdeltafr/2, CDdeltae/2, CDq/2, CDalpha_dot/2, CDalpha/2  "<beta>"
  CDalpha/1 -> Product/1

== system mainV03_56/LIBIS Plant/Aerodynamics/CL ==
  prelook-ups : Inport
  plantData : Inport  Port=2
  actuators : Inport  Port=3
  Add1 : Sum  Inputs=+++++++
  Bus Selector2 : BusSelector  OutputSignals=alpha,alpha_dot,Omega_body.q
  Bus Selector4 : BusSelector  OutputSignals=alpha,beta,alt,xcg,deltae,deltar,deltafr,deltafl
  Bus Selector5 : BusSelector  OutputSignals=deltae,deltafr,deltafl
  CL0 : Interpolation_n-D  NumberOfTableDimensions=8  Table=LD.Stability.CL0  RequireIndexFractionAsBus=on  InternalRulePriority=Speed
      settings: InputPortMap=u0,u1,u2,u3,u4,u5,u6,u7
  CLalpha : Interpolation_n-D  NumberOfTableDimensions=8  Table=LD.Stability.CLalpha  ExtrapMethod=Clip  DiagnosticForOutOfRangeInput=Warning  RequireIndexFractionAsBus=on  ValidIndexMayReachLast=on  InternalRulePriority=Speed
      settings: InputPortMap=u0,u1,u2,u3,u4,u5,u6,u7
  CLalpha_dot : Interpolation_n-D  NumberOfTableDimensions=8  Table=LD.Stability.CLalpha_dot  ExtrapMethod=Clip  RequireIndexFractionAsBus=on  ValidIndexMayReachLast=on  InternalRulePriority=Speed
      settings: InputPortMap=u0,u1,u2,u3,u4,u5,u6,u7
  CLdeltae : Interpolation_n-D  NumberOfTableDimensions=8  Table=LD.Stability.CLdeltae  ExtrapMethod=Clip  RequireIndexFractionAsBus=on  ValidIndexMayReachLast=on  InternalRulePriority=Speed
      settings: InputPortMap=u0,u1,u2,u3,u4,u5,u6,u7
  CLdeltafr : Interpolation_n-D  NumberOfTableDimensions=8  Table=LD.Stability.CLdeltafr  ExtrapMethod=Clip  RequireIndexFractionAsBus=on  ValidIndexMayReachLast=on  InternalRulePriority=Speed
      settings: InputPortMap=u0,u1,u2,u3,u4,u5,u6,u7
  CLdeltafrl : Interpolation_n-D  NumberOfTableDimensions=8  Table=LD.Stability.CLdeltafl  ExtrapMethod=Clip  RequireIndexFractionAsBus=on  ValidIndexMayReachLast=on  InternalRulePriority=Speed
      settings: InputPortMap=u0,u1,u2,u3,u4,u5,u6,u7
  CLq : Interpolation_n-D  NumberOfTableDimensions=8  Table=LD.Stability.CLq  ExtrapMethod=Clip  RequireIndexFractionAsBus=on  ValidIndexMayReachLast=on  InternalRulePriority=Speed
      settings: InputPortMap=u0,u1,u2,u3,u4,u5,u6,u7
  Product{6..11} (6 alike) : Product
  CL : Outport
  wires:
  prelook-ups/1 -> Bus Selector4/1
  CL0/1 -> Add1/1
  Add1/1 -> CL/1
  plantData/1 -> Bus Selector2/1
  actuators/1 -> Bus Selector5/1
  Product6/1 -> Add1/2
  Bus Selector2/1 -> Product6/2  "<alpha>"
  Bus Selector5/1 -> Product9/2  "<deltae>"
  CLdeltae/1 -> Product9/1
  Product9/1 -> Add1/5
  Product8/1 -> Add1/4
  Product7/1 -> Add1/3
  CLalpha_dot/1 -> Product7/1
  CLq/1 -> Product8/1
  Bus Selector2/3 -> Product8/2  "<q>"
  Bus Selector2/2 -> Product7/2  "<alpha_dot>"
  Bus Selector4/8 -> CL0/8, CLalpha/8, CLq/8, CLdeltafrl/8, CLdeltafr/8, CLdeltae/8, CLalpha_dot/8  "<deltafl>"
  Bus Selector4/7 -> CL0/7, CLalpha/7, CLq/7, CLdeltafrl/7, CLdeltafr/7, CLdeltae/7, CLalpha_dot/7  "<deltafr>"
  Bus Selector4/6 -> CL0/6, CLalpha/6, CLq/6, CLdeltafrl/6, CLdeltafr/6, CLdeltae/6, CLalpha_dot/6  "<deltar>"
  Bus Selector4/5 -> CL0/5, CLalpha/5, CLq/5, CLdeltafrl/5, CLdeltafr/5, CLdeltae/5, CLalpha_dot/5  "<deltae>"
  Bus Selector4/3 -> CL0/3, CLalpha/3, CLq/3, CLdeltafrl/3, CLdeltafr/3, CLdeltae/3, CLalpha_dot/3  "<alt>"
  Bus Selector4/4 -> CL0/4, CLalpha/4, CLq/4, CLdeltafrl/4, CLdeltafr/4, CLdeltae/4, CLalpha_dot/4  "<xcg>"
  Bus Selector4/1 -> CL0/1, CLalpha/1, CLdeltafrl/1, CLdeltafr/1, CLdeltae/1, CLq/1, CLalpha_dot/1  "<alpha>"
  Bus Selector5/3 -> Product11/2  "<deltafl>"
  CLdeltafrl/1 -> Product11/1
  Product11/1 -> Add1/7
  Product10/1 -> Add1/6
  CLdeltafr/1 -> Product10/1
  Bus Selector5/2 -> Product10/2  "<deltafr>"
  Bus Selector4/2 -> CL0/2, CLdeltafrl/2, CLdeltafr/2, CLdeltae/2, CLq/2, CLalpha_dot/2, CLalpha/2  "<beta>"
  CLalpha/1 -> Product6/1

== system mainV03_56/LIBIS Plant/Aerodynamics/CY ==
  prelook-ups : Inport
  plantData : Inport  Port=2
  actuators : Inport  Port=3
  Add : Sum  Inputs=++++++
  Bus Selector : BusSelector  OutputSignals=beta,Omega_body.p,Omega_body.r
  Bus Selector1 : BusSelector  OutputSignals=alpha,beta,alt,xcg,deltae,deltar,deltafr,deltafl
  Bus Selector2 : BusSelector  OutputSignals=deltar,deltafr,deltafl
  CYbeta : Interpolation_n-D  NumberOfTableDimensions=8  Table=LD.Stability.CYbeta  ExtrapMethod=Clip  RequireIndexFractionAsBus=on  ValidIndexMayReachLast=on  InternalRulePriority=Speed
      settings: InputPortMap=u0,u1,u2,u3,u4,u5,u6,u7
  CYdeltafl : Interpolation_n-D  NumberOfTableDimensions=8  Table=LD.Stability.CYdeltafl  ExtrapMethod=Clip  RequireIndexFractionAsBus=on  ValidIndexMayReachLast=on  InternalRulePriority=Speed
      settings: InputPortMap=u0,u1,u2,u3,u4,u5,u6,u7
  CYdeltafr : Interpolation_n-D  NumberOfTableDimensions=8  Table=LD.Stability.CYdeltafr  ExtrapMethod=Clip  RequireIndexFractionAsBus=on  ValidIndexMayReachLast=on  InternalRulePriority=Speed
      settings: InputPortMap=u0,u1,u2,u3,u4,u5,u6,u7
  "CYdeltar " : Interpolation_n-D  NumberOfTableDimensions=8  Table=LD.Stability.CYdeltar  ExtrapMethod=Clip  RequireIndexFractionAsBus=on  ValidIndexMayReachLast=on  InternalRulePriority=Speed
      settings: InputPortMap=u0,u1,u2,u3,u4,u5,u6,u7
  CYp : Interpolation_n-D  NumberOfTableDimensions=8  Table=LD.Stability.CYp  ExtrapMethod=Clip  RequireIndexFractionAsBus=on  ValidIndexMayReachLast=on  InternalRulePriority=Speed
      settings: InputPortMap=u0,u1,u2,u3,u4,u5,u6,u7
  CYr : Interpolation_n-D  NumberOfTableDimensions=8  Table=LD.Stability.CYr  ExtrapMethod=Clip  RequireIndexFractionAsBus=on  ValidIndexMayReachLast=on  InternalRulePriority=Speed
      settings: InputPortMap=u0,u1,u2,u3,u4,u5,u6,u7
  Product{,1..5} (6 alike) : Product
  CY : Outport
  wires:
  Bus Selector1/8 -> CYbeta/8, CYr/8, "CYdeltar "/8, CYdeltafl/8, CYdeltafr/8, CYp/8  "<deltafl>"
  Bus Selector1/7 -> CYbeta/7, CYr/7, "CYdeltar "/7, CYdeltafl/7, CYdeltafr/7, CYp/7  "<deltafr>"
  Bus Selector1/6 -> CYbeta/6, CYr/6, "CYdeltar "/6, CYdeltafl/6, CYdeltafr/6, CYp/6  "<deltar>"
  prelook-ups/1 -> Bus Selector1/1
  Bus Selector1/5 -> CYbeta/5, CYr/5, "CYdeltar "/5, CYdeltafl/5, CYdeltafr/5, CYp/5  "<deltae>"
  Bus Selector1/3 -> CYbeta/3, CYr/3, "CYdeltar "/3, CYdeltafl/3, CYdeltafr/3, CYp/3  "<alt>"
  Bus Selector1/4 -> CYbeta/4, CYr/4, "CYdeltar "/4, CYdeltafl/4, CYdeltafr/4, CYp/4  "<xcg>"
  Bus Selector1/1 -> CYbeta/1, CYdeltafl/1, CYdeltafr/1, "CYdeltar "/1, CYr/1, CYp/1  "<alpha>"
  Add/1 -> CY/1
  plantData/1 -> Bus Selector/1
  actuators/1 -> Bus Selector2/1
  CYbeta/1 -> Product/1
  Product/1 -> Add/1
  Bus Selector/1 -> Product/2  "<beta>"
  Bus Selector2/1 -> Product3/2  "<deltar>"
  "CYdeltar "/1 -> Product3/1
  Product3/1 -> Add/4
  Product2/1 -> Add/3
  Product1/1 -> Add/2
  CYp/1 -> Product1/1
  CYr/1 -> Product2/1
  Bus Selector/3 -> Product2/2  "<r>"
  Bus Selector/2 -> Product1/2  "<p>"
  CYdeltafl/1 -> Product5/1
  Product5/1 -> Add/6
  Product4/1 -> Add/5
  CYdeltafr/1 -> Product4/1
  Bus Selector2/2 -> Product4/2  "<deltafr>"
  Bus Selector2/3 -> Product5/2  "<deltafl>"
  Bus Selector1/2 -> CYdeltafl/2, CYdeltafr/2, "CYdeltar "/2, CYr/2, CYp/2, CYbeta/2  "<beta>"

== system mainV03_56/LIBIS Plant/Aerodynamics/Cl ==
  prelook-ups1 : Inport
  plantData : Inport  Port=2
  actuators : Inport  Port=3
  Add1 : Sum  Inputs=++++++
  Bus Selector3 : BusSelector  OutputSignals=beta,Omega_body.p,Omega_body.r
  Bus Selector4 : BusSelector  OutputSignals=alpha,beta,alt,xcg,deltae,deltar,deltafr,deltafl
  Bus Selector5 : BusSelector  OutputSignals=deltar,deltafr,deltafl
  Clbeta : Interpolation_n-D  NumberOfTableDimensions=8  Table=LD.Stability.Clbeta  ExtrapMethod=Clip  RequireIndexFractionAsBus=on  ValidIndexMayReachLast=on  InternalRulePriority=Speed
      settings: InputPortMap=u0,u1,u2,u3,u4,u5,u6,u7
  Cldeltafl : Interpolation_n-D  NumberOfTableDimensions=8  Table=LD.Stability.Cldeltafl  ExtrapMethod=Clip  RequireIndexFractionAsBus=on  ValidIndexMayReachLast=on  InternalRulePriority=Speed
      settings: InputPortMap=u0,u1,u2,u3,u4,u5,u6,u7
  Cldeltafr : Interpolation_n-D  NumberOfTableDimensions=8  Table=LD.Stability.Cldeltafr  ExtrapMethod=Clip  RequireIndexFractionAsBus=on  ValidIndexMayReachLast=on  InternalRulePriority=Speed
      settings: InputPortMap=u0,u1,u2,u3,u4,u5,u6,u7
  "Cldeltar " : Interpolation_n-D  NumberOfTableDimensions=8  Table=LD.Stability.Cldeltar  ExtrapMethod=Clip  RequireIndexFractionAsBus=on  ValidIndexMayReachLast=on  InternalRulePriority=Speed
      settings: InputPortMap=u0,u1,u2,u3,u4,u5,u6,u7
  Clp : Interpolation_n-D  NumberOfTableDimensions=8  Table=LD.Stability.Clp  ExtrapMethod=Clip  RequireIndexFractionAsBus=on  ValidIndexMayReachLast=on  InternalRulePriority=Speed
      settings: InputPortMap=u0,u1,u2,u3,u4,u5,u6,u7
  Clr : Interpolation_n-D  NumberOfTableDimensions=8  Table=LD.Stability.Clr  ExtrapMethod=Clip  RequireIndexFractionAsBus=on  ValidIndexMayReachLast=on  InternalRulePriority=Speed
      settings: InputPortMap=u0,u1,u2,u3,u4,u5,u6,u7
  Product{6..11} (6 alike) : Product
  Cl : Outport
  wires:
  Bus Selector4/8 -> Clbeta/8, Clr/8, "Cldeltar "/8, Cldeltafl/8, Cldeltafr/8, Clp/8  "<deltafl>"
  Bus Selector4/7 -> Clbeta/7, Clr/7, "Cldeltar "/7, Cldeltafl/7, Cldeltafr/7, Clp/7  "<deltafr>"
  Bus Selector4/6 -> Clbeta/6, Clr/6, "Cldeltar "/6, Cldeltafl/6, Cldeltafr/6, Clp/6  "<deltar>"
  prelook-ups1/1 -> Bus Selector4/1
  Bus Selector4/5 -> Clbeta/5, Clr/5, "Cldeltar "/5, Cldeltafl/5, Cldeltafr/5, Clp/5  "<deltae>"
  Bus Selector4/3 -> Clbeta/3, Clr/3, "Cldeltar "/3, Cldeltafl/3, Cldeltafr/3, Clp/3  "<alt>"
  Bus Selector4/4 -> Clbeta/4, Clr/4, "Cldeltar "/4, Cldeltafl/4, Cldeltafr/4, Clp/4  "<xcg>"
  Bus Selector4/1 -> Clbeta/1, Cldeltafl/1, Cldeltafr/1, "Cldeltar "/1, Clr/1, Clp/1  "<alpha>"
  Add1/1 -> Cl/1
  plantData/1 -> Bus Selector3/1
  actuators/1 -> Bus Selector5/1
  Clbeta/1 -> Product6/1
  Product6/1 -> Add1/1
  Bus Selector3/1 -> Product6/2  "<beta>"
  Bus Selector5/1 -> Product9/2  "<deltar>"
  "Cldeltar "/1 -> Product9/1
  Product9/1 -> Add1/4
  Product8/1 -> Add1/3
  Product7/1 -> Add1/2
  Clp/1 -> Product7/1
  Clr/1 -> Product8/1
  Bus Selector3/3 -> Product8/2  "<r>"
  Bus Selector3/2 -> Product7/2  "<p>"
  Cldeltafl/1 -> Product11/1
  Product11/1 -> Add1/6
  Product10/1 -> Add1/5
  Cldeltafr/1 -> Product10/1
  Bus Selector5/2 -> Product10/2  "<deltafr>"
  Bus Selector5/3 -> Product11/2  "<deltafl>"
  Bus Selector4/2 -> Cldeltafl/2, Cldeltafr/2, "Cldeltar "/2, Clr/2, Clp/2, Clbeta/2  "<beta>"

== system mainV03_56/LIBIS Plant/Aerodynamics/Cm ==
  prelook-ups : Inport
  plantData : Inport  Port=2
  actuators : Inport  Port=3
  Add2 : Sum  Inputs=+++++++
  Bus Selector2 : BusSelector  OutputSignals=alpha,alpha_dot,Omega_body.q
  Bus Selector4 : BusSelector  OutputSignals=alpha,beta,alt,xcg,deltae,deltar,deltafr,deltafl
  Bus Selector5 : BusSelector  OutputSignals=deltae,deltafr,deltafl
  Cm0 : Interpolation_n-D  NumberOfTableDimensions=8  Table=LD.Stability.Cm0  RequireIndexFractionAsBus=on  InternalRulePriority=Speed
      settings: InputPortMap=u0,u1,u2,u3,u4,u5,u6,u7
  Cmalpha : Interpolation_n-D  NumberOfTableDimensions=8  Table=LD.Stability.Cmalpha  ExtrapMethod=Clip  RequireIndexFractionAsBus=on  ValidIndexMayReachLast=on  InternalRulePriority=Speed
      settings: InputPortMap=u0,u1,u2,u3,u4,u5,u6,u7
  Cmalpha_dot : Interpolation_n-D  NumberOfTableDimensions=8  Table=LD.Stability.Cmalpha_dot  ExtrapMethod=Clip  RequireIndexFractionAsBus=on  ValidIndexMayReachLast=on  InternalRulePriority=Speed
      settings: InputPortMap=u0,u1,u2,u3,u4,u5,u6,u7
  Cmdeltae : Interpolation_n-D  NumberOfTableDimensions=8  Table=LD.Stability.Cmdeltae  ExtrapMethod=Clip  RequireIndexFractionAsBus=on  ValidIndexMayReachLast=on  InternalRulePriority=Speed
      settings: InputPortMap=u0,u1,u2,u3,u4,u5,u6,u7
  Cmdeltafl : Interpolation_n-D  NumberOfTableDimensions=8  Table=LD.Stability.CLdeltafl  ExtrapMethod=Clip  RequireIndexFractionAsBus=on  ValidIndexMayReachLast=on  InternalRulePriority=Speed
      settings: InputPortMap=u0,u1,u2,u3,u4,u5,u6,u7
  Cmdeltafr : Interpolation_n-D  NumberOfTableDimensions=8  Table=LD.Stability.Cmdeltafr  ExtrapMethod=Clip  RequireIndexFractionAsBus=on  ValidIndexMayReachLast=on  InternalRulePriority=Speed
      settings: InputPortMap=u0,u1,u2,u3,u4,u5,u6,u7
  Cmq : Interpolation_n-D  NumberOfTableDimensions=8  Table=LD.Stability.Cmq  ExtrapMethod=Clip  RequireIndexFractionAsBus=on  ValidIndexMayReachLast=on  InternalRulePriority=Speed
      settings: InputPortMap=u0,u1,u2,u3,u4,u5,u6,u7
  Product{6..11} (6 alike) : Product
  Cm : Outport
  wires:
  prelook-ups/1 -> Bus Selector4/1
  Cm0/1 -> Add2/1
  Add2/1 -> Cm/1
  plantData/1 -> Bus Selector2/1
  actuators/1 -> Bus Selector5/1
  Product6/1 -> Add2/2
  Bus Selector2/1 -> Product6/2  "<alpha>"
  Bus Selector5/1 -> Product9/2  "<deltae>"
  Cmdeltae/1 -> Product9/1
  Product9/1 -> Add2/5
  Product8/1 -> Add2/4
  Product7/1 -> Add2/3
  Cmalpha_dot/1 -> Product7/1
  Cmq/1 -> Product8/1
  Bus Selector2/3 -> Product8/2  "<q>"
  Bus Selector2/2 -> Product7/2  "<alpha_dot>"
  Bus Selector4/8 -> Cm0/8, Cmalpha/8, Cmq/8, Cmdeltafl/8, Cmdeltafr/8, Cmdeltae/8, Cmalpha_dot/8  "<deltafl>"
  Bus Selector4/7 -> Cm0/7, Cmalpha/7, Cmq/7, Cmdeltafl/7, Cmdeltafr/7, Cmdeltae/7, Cmalpha_dot/7  "<deltafr>"
  Bus Selector4/6 -> Cm0/6, Cmalpha/6, Cmq/6, Cmdeltafl/6, Cmdeltafr/6, Cmdeltae/6, Cmalpha_dot/6  "<deltar>"
  Bus Selector4/5 -> Cm0/5, Cmalpha/5, Cmq/5, Cmdeltafl/5, Cmdeltafr/5, Cmdeltae/5, Cmalpha_dot/5  "<deltae>"
  Bus Selector4/3 -> Cm0/3, Cmalpha/3, Cmq/3, Cmdeltafl/3, Cmdeltafr/3, Cmdeltae/3, Cmalpha_dot/3  "<alt>"
  Bus Selector4/4 -> Cm0/4, Cmalpha/4, Cmq/4, Cmdeltafl/4, Cmdeltafr/4, Cmdeltae/4, Cmalpha_dot/4  "<xcg>"
  Bus Selector4/1 -> Cm0/1, Cmalpha/1, Cmdeltafl/1, Cmdeltafr/1, Cmdeltae/1, Cmq/1, Cmalpha_dot/1  "<alpha>"
  Bus Selector5/3 -> Product11/2  "<deltafl>"
  Cmdeltafl/1 -> Product11/1
  Product11/1 -> Add2/7
  Product10/1 -> Add2/6
  Cmdeltafr/1 -> Product10/1
  Bus Selector5/2 -> Product10/2  "<deltafr>"
  Bus Selector4/2 -> Cm0/2, Cmdeltafl/2, Cmdeltafr/2, Cmdeltae/2, Cmq/2, Cmalpha_dot/2, Cmalpha/2  "<beta>"
  Cmalpha/1 -> Product6/1

== system mainV03_56/LIBIS Plant/Aerodynamics/Cn ==
  prelook-ups : Inport
  plantData : Inport  Port=2
  actuators : Inport  Port=3
  Add1 : Sum  Inputs=++++++
  Bus Selector3 : BusSelector  OutputSignals=beta,Omega_body.p,Omega_body.r
  Bus Selector4 : BusSelector  OutputSignals=alpha,beta,alt,xcg,deltae,deltar,deltafr,deltafl
  Bus Selector5 : BusSelector  OutputSignals=deltar,deltafr,deltafl
  Cnbeta : Interpolation_n-D  NumberOfTableDimensions=8  Table=LD.Stability.Cnbeta  ExtrapMethod=Clip  RequireIndexFractionAsBus=on  ValidIndexMayReachLast=on  InternalRulePriority=Speed
      settings: InputPortMap=u0,u1,u2,u3,u4,u5,u6,u7
  Cndeltafl : Interpolation_n-D  NumberOfTableDimensions=8  Table=LD.Stability.Cndeltafl  ExtrapMethod=Clip  RequireIndexFractionAsBus=on  ValidIndexMayReachLast=on  InternalRulePriority=Speed
      settings: InputPortMap=u0,u1,u2,u3,u4,u5,u6,u7
  Cndeltafr : Interpolation_n-D  NumberOfTableDimensions=8  Table=LD.Stability.Cndeltafr  ExtrapMethod=Clip  RequireIndexFractionAsBus=on  ValidIndexMayReachLast=on  InternalRulePriority=Speed
      settings: InputPortMap=u0,u1,u2,u3,u4,u5,u6,u7
  "Cndeltar " : Interpolation_n-D  NumberOfTableDimensions=8  Table=LD.Stability.Cndeltar  ExtrapMethod=Clip  RequireIndexFractionAsBus=on  ValidIndexMayReachLast=on  InternalRulePriority=Speed
      settings: InputPortMap=u0,u1,u2,u3,u4,u5,u6,u7
  Cnp : Interpolation_n-D  NumberOfTableDimensions=8  Table=LD.Stability.Cnp  ExtrapMethod=Clip  RequireIndexFractionAsBus=on  ValidIndexMayReachLast=on  InternalRulePriority=Speed
      settings: InputPortMap=u0,u1,u2,u3,u4,u5,u6,u7
  Cnr : Interpolation_n-D  NumberOfTableDimensions=8  Table=LD.Stability.Cnr  ExtrapMethod=Clip  RequireIndexFractionAsBus=on  ValidIndexMayReachLast=on  InternalRulePriority=Speed
      settings: InputPortMap=u0,u1,u2,u3,u4,u5,u6,u7
  Product{6..11} (6 alike) : Product
  Cn : Outport
  wires:
  Bus Selector4/8 -> Cnbeta/8, Cnr/8, "Cndeltar "/8, Cndeltafl/8, Cndeltafr/8, Cnp/8  "<deltafl>"
  Bus Selector4/7 -> Cnbeta/7, Cnr/7, "Cndeltar "/7, Cndeltafl/7, Cndeltafr/7, Cnp/7  "<deltafr>"
  Bus Selector4/6 -> Cnbeta/6, Cnr/6, "Cndeltar "/6, Cndeltafl/6, Cndeltafr/6, Cnp/6  "<deltar>"
  prelook-ups/1 -> Bus Selector4/1
  Bus Selector4/5 -> Cnbeta/5, Cnr/5, "Cndeltar "/5, Cndeltafl/5, Cndeltafr/5, Cnp/5  "<deltae>"
  Bus Selector4/3 -> Cnbeta/3, Cnr/3, "Cndeltar "/3, Cndeltafl/3, Cndeltafr/3, Cnp/3  "<alt>"
  Bus Selector4/4 -> Cnbeta/4, Cnr/4, "Cndeltar "/4, Cndeltafl/4, Cndeltafr/4, Cnp/4  "<xcg>"
  Bus Selector4/1 -> Cnbeta/1, Cndeltafl/1, Cndeltafr/1, "Cndeltar "/1, Cnr/1, Cnp/1  "<alpha>"
  Add1/1 -> Cn/1
  plantData/1 -> Bus Selector3/1
  actuators/1 -> Bus Selector5/1
  Cnbeta/1 -> Product6/1
  Product6/1 -> Add1/1
  Bus Selector3/1 -> Product6/2  "<beta>"
  Bus Selector5/1 -> Product9/2  "<deltar>"
  "Cndeltar "/1 -> Product9/1
  Product9/1 -> Add1/4
  Product8/1 -> Add1/3
  Product7/1 -> Add1/2
  Cnp/1 -> Product7/1
  Cnr/1 -> Product8/1
  Bus Selector3/3 -> Product8/2  "<r>"
  Bus Selector3/2 -> Product7/2  "<p>"
  Cndeltafl/1 -> Product11/1
  Product11/1 -> Add1/6
  Product10/1 -> Add1/5
  Cndeltafr/1 -> Product10/1
  Bus Selector5/2 -> Product10/2  "<deltafr>"
  Bus Selector5/3 -> Product11/2  "<deltafl>"
  Bus Selector4/2 -> Cndeltafl/2, Cndeltafr/2, "Cndeltar "/2, Cnr/2, Cnp/2, Cnbeta/2  "<beta>"

== system mainV03_56/LIBIS Plant/Propulsion/8S 25C Battery ==
  note: Hay 2 baterías en paralelo
  note: https://www.maxamps.com/lipo-11000-8s-29-6v-battery-pack
  note: 11,000mah capacity
      | 8S 29.6 volts
      | True 40C rating
      | Lifetime warranty
      | 5C fast charge capable
      | 100% waterproof
      | Built today with factory fresh cells
      | Built with genuine 12awg Deans Ultra wire
      | We add the connector and JST-XH balancing tap for you
      | 158mm x 59mm x 81mm, 1690g
  note: MaxAmps LiPo 11,000 8S 29.6v Battery Pack
  Battery_Capacity : Constant  Value=22
  Battery_Voltage : Constant  Value=29.6
  Max_discharge_rate : Constant  Value=440
  profundidad_descarga : Constant  Value=0.95
  rendimiento_bateria : Constant  Value=0.98
  C_battery : Outport  Unit=A*h
  deep_discharge_battery : Outport  Port=2  Unit=1
  V_battery : Outport  Port=3  Unit=V
  eta_battery : Outport  Port=4  Unit=1
  max_discharge_rate : Outport  Port=5  Unit=A*h
  wires:
  Battery_Voltage/1 -> V_battery/1
  Battery_Capacity/1 -> C_battery/1
  profundidad_descarga/1 -> deep_discharge_battery/1
  rendimiento_bateria/1 -> eta_battery/1
  Max_discharge_rate/1 -> max_discharge_rate/1

== system mainV03_56/LIBIS Plant/Propulsion/Variant_Motor_1 ==
  note: 1) Add Subsystem or Model blocks as valid variant choices.
      | 2) You cannot connect blocks at this level. At simulation, connectivity is automatically
      | determined, based on the active variant and port name matching.
  Vbattery : Inport
  Throttle : Inport  Port=2
  envData : Inport  Port=3
  plantData : Inport  Port=4
  mappedMotor_1 : Subsystem  VariantControl=mappedMotors==1
  noMappedMotor_1 : Subsystem  VariantControl=mappedMotors~=1
  Im : Outport
  Thrust : Outport  Port=2
  Thrust_moment : Outport  Port=3

== system mainV03_56/LIBIS Plant/Propulsion/Variant_Motor_2 ==
  note: 1) Add Subsystem or Model blocks as valid variant choices.
      | 2) You cannot connect blocks at this level. At simulation, connectivity is automatically
      | determined, based on the active variant and port name matching.
  Vbattery : Inport
  Throttle : Inport  Port=2
  envData : Inport  Port=3
  plantData : Inport  Port=4
  mappedMotor_2 : Subsystem  VariantControl=mappedMotors==1
  noMappedMotor_2 : Subsystem  VariantControl=mappedMotors~=1
  Im : Outport
  Thrust : Outport  Port=2
  Thrust_moment : Outport  Port=3

== system mainV03_56/LIBIS Plant/Propulsion/Variant_Motor_3 ==
  note: 1) Add Subsystem or Model blocks as valid variant choices.
      | 2) You cannot connect blocks at this level. At simulation, connectivity is automatically
      | determined, based on the active variant and port name matching.
  Vbattery : Inport
  Throttle : Inport  Port=2
  envData : Inport  Port=3
  plantData : Inport  Port=4
  mappedMotor_3 : Subsystem  VariantControl=mappedMotors==1
  noMappedMotor_3 : Subsystem  VariantControl=mappedMotors~=1
  Im : Outport
  Thrust : Outport  Port=2
  Thrust_moment : Outport  Port=3
